simulink library "ctrlAllocMatrix_cl"  (R2018b)
settings: Solver=VariableStepAuto  StartTime=0.0  StopTime=10.0  RelTol=1e-3
undefined symbols (not defined in the file or in its folder): aeroStruct
libraries: vrlib x3, vectorNormalizer_ul x2, linearLeastSqrs_ul x1, dynamicPressure_ul x1, alphaBeta_ul x1, localApparentWind_ul x1
settings Model: Creator=mcobb  LastModifiedBy=James Reed

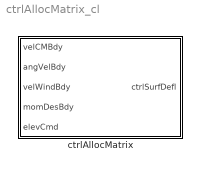
== system ctrlAllocMatrix_cl ==
  ctrlAllocMatrix : Subsystem  mask{aeroStruct=aeroStruct, fluidDensity=0, ctrlUpMax=0, ctrlDnMax=0}
      mask prompts: aeroStruct "Aerodynamic surface structure"; fluidDensity "Fluid density"; ctrlUpMax "Max Up Ctrl Surf Defl"; ctrlDnMax "Max Down Ctrl Surf Defl"
      mask TypeOptions aeroStruct: momentComponentVector/aeroStruct
      mask TypeOptions fluidDensity: momentComponentVector/fluidDensity

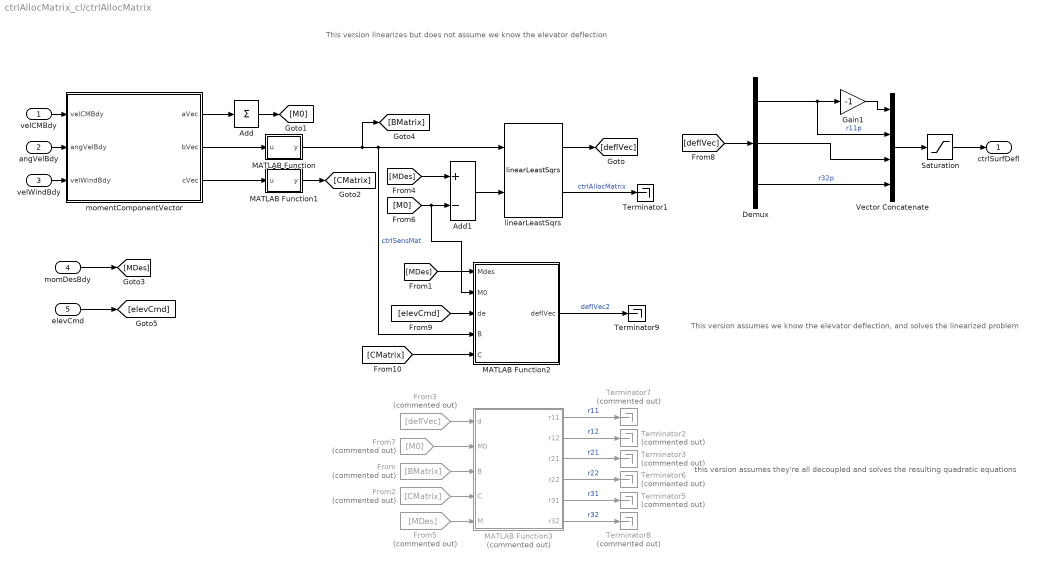
== system ctrlAllocMatrix_cl/ctrlAllocMatrix ==
  note: This version linearizes but does not assume we know the elevator deflection
  note: this version assumes they're all decoupled and solves the resulting quadratic equations
  note: This version assumes we know the elevator deflection, and solves the linearized problem
  velCMBdy : Inport
  angVelBdy : Inport  Port=2
  velWindBdy : Inport  Port=3
  momDesBdy : Inport  Port=4
  elevCmd : Inport  Port=5
  Add : Sum  Inputs=+  CollapseMode=Specified dimension  CollapseDim=2
  Add1 : Sum  Inputs=+-
  Demux : Demux  Outputs=3
  From : From  Commented=on  GotoTag=BMatrix
  From2 : From  Commented=on  GotoTag=CMatrix
  From3 : From  Commented=on  GotoTag=deflVec
  From5 : From  Commented=on  GotoTag=MDes
  From7 : From  Commented=on  GotoTag=M0
  Gain1 : Gain  Gain=-1
  MATLAB Function : MATLAB Function  TreatAsAtomicUnit=on
  MATLAB Function1 : MATLAB Function  TreatAsAtomicUnit=on
  MATLAB Function2 : MATLAB Function  TreatAsAtomicUnit=on
  MATLAB Function3 : MATLAB Function  Commented=on  TreatAsAtomicUnit=on
  Saturation : Saturate  UpperLimit=ctrlUpMax  LowerLimit=ctrlDnMax
  Terminator1 : Terminator
  Terminator{2..3,5..8} (6 alike) : Terminator  Commented=on
  Terminator9 : Terminator
  Vector Concatenate : Concatenate  NumInputs=4
  linearLeastSqrs : linearLeastSqrs_ul/linearLeastSqrs  SystemSampleTime=-1
  momentComponentVector : Subsystem  mask{aeroStruct=aeroStruct, fluidDensity=fluidDensity}
      mask prompts: aeroStruct "Aerodynamic surface structure"; fluidDensity "Fluid density"
      mask help:
      | Input must be an 1×N struct array with fields:
      |     refArea
      |     aeroCentPosVec
      |     spanUnitVec
      |     chordUnitVec
      |     CL
      |     CD
      |     alpha
      |     GainCL
      |     GainCD
      |
      | where N is the number of aerodynamic surfaces
  ctrlSurfDefl : Outport
  wires:
  velWindBdy/1 -> momentComponentVector/3(velWindBdy)
  velCMBdy/1 -> momentComponentVector/1(velCMBdy)
  angVelBdy/1 -> momentComponentVector/2(angVelBdy)
  momentComponentVector/1(aVec) -> Add/1
  momentComponentVector/3(cVec) -> MATLAB Function1/1(u)
  Add/1 -> [M0]
  momDesBdy/1 -> [MDes]
  [M0] -> MATLAB Function2/2(M0), Add1/2
  Add1/1 -> linearLeastSqrs/2
  MATLAB Function/1(y) -> [BMatrix], MATLAB Function2/4(B), linearLeastSqrs/1  "ctrlSensMat"
  linearLeastSqrs/1 -> [deflVec]
  momentComponentVector/2(bVec) -> MATLAB Function/1(u)
  Demux/2 -> Vector Concatenate/3
  Demux/1 -> Vector Concatenate/2, Gain1/1  "r11p"
  Vector Concatenate/1 -> Saturation/1
  Saturation/1 -> ctrlSurfDefl/1
  Gain1/1 -> Vector Concatenate/1
  linearLeastSqrs/2 -> Terminator1/1  "ctrlAllocMatrix"
  MATLAB Function1/1(y) -> [CMatrix]
  [MDes] -> Add1/1
  Demux/3 -> Vector Concatenate/4  "r32p"
  From2/1 -> MATLAB Function3/4(C)
  From3/1 -> MATLAB Function3/1(d)
  From5/1 -> MATLAB Function3/5(M)
  From7/1 -> MATLAB Function3/2(M0)
  From/1 -> MATLAB Function3/3(B)
  MATLAB Function3/2(r12) -> Terminator2/1  "r12"
  MATLAB Function3/3(r21) -> Terminator3/1  "r21"
  MATLAB Function3/5(r31) -> Terminator5/1  "r31"
  MATLAB Function3/6(r32) -> Terminator8/1  "r32"
  MATLAB Function3/4(r22) -> Terminator6/1  "r22"
  MATLAB Function3/1(r11) -> Terminator7/1  "r11"
  elevCmd/1 -> [elevCmd]
  [MDes] -> MATLAB Function2/1(Mdes)
  [elevCmd] -> MATLAB Function2/3(de)
  [CMatrix] -> MATLAB Function2/5(C)
  MATLAB Function2/1(deflVec) -> Terminator9/1  "deflVec2"
  [deflVec] -> Demux/1

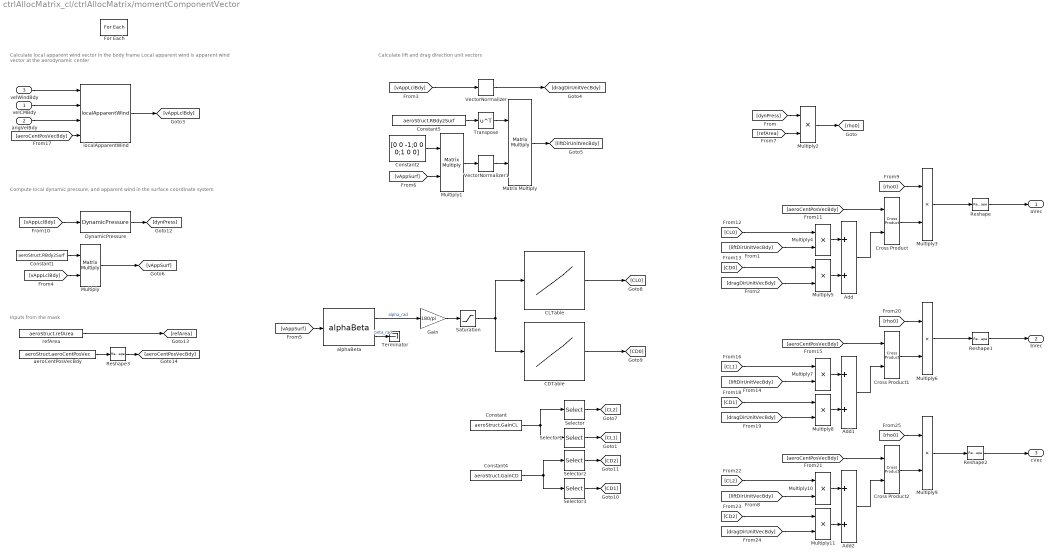
== system ctrlAllocMatrix_cl/ctrlAllocMatrix/momentComponentVector ==
  note: Compute local dynamic pressure,
      | and apparent wind in the surface coordinate system
  note: Inputs from the mask
  note: Calculate lift and drag direction unit vectors
  note: Calculate local apparent wind vector in the body frame
      | Local apparent wind is apparent wind vector at the aerodynamic center
  velCMBdy : Inport
  angVelBdy : Inport  Port=2
  velWindBdy : Inport  Port=3
  Add : Sum
  Add1 : Sum
  Add2 : Sum
  CDTable : Lookup_n-D  NumberOfTableDimensions=1  LookupTableObject=CLTable  BreakpointsForDimension1=aeroStruct.alpha  Table=aeroStruct.CD  ExtrapMethod=Clip  UseLastTableValue=on  InternalRulePriority=Speed  RndMeth=Simplest  InputSameDT=on
  CLTable : Lookup_n-D  NumberOfTableDimensions=1  LookupTableObject=CLTable  BreakpointsForDimension1=aeroStruct.alpha  Table=aeroStruct.CL  ExtrapMethod=Clip  UseLastTableValue=on  InternalRulePriority=Speed  RndMeth=Simplest  InputSameDT=on
  Constant : Constant  Value=aeroStruct.GainCL
  Constant1 : Constant  Value=aeroStruct.RBdy2Surf
  Constant2 : Constant  Value=[0 0 -1;0 0 0;1 0 0]
  Constant4 : Constant  Value=aeroStruct.GainCD
  Constant5 : Constant  Value=aeroStruct.RBdy2Surf
  Cross Product : vrlib/Utilities/Cross Product
      settings: SourceProductBaseCode=VR
  Cross Product1 : vrlib/Utilities/Cross Product
      settings: SourceProductBaseCode=VR
  Cross Product2 : vrlib/Utilities/Cross Product
      settings: SourceProductBaseCode=VR
  DynamicPressure : dynamicPressure_ul/DynamicPressure  rho=fluidDensity
  For Each : ForEach  DisableCoverage=on  IterateSubsysMaskParameter=on,off  SubsysMaskParameterIterationDimension=2,1  IndexMode=One-based
  Gain : Gain  Gain=180/pi
  Matrix Multiply : Product  Multiplication=Matrix(*)
  Multiply : Product  Multiplication=Matrix(*)
  Multiply1 : Product  Multiplication=Matrix(*)
  Multiply{2..11} (10 alike) : Product
  Reshape{,1..3} (4 alike) : Reshape  OutputDimensionality=Column vector (2-D)
  Saturation : Saturate  UpperLimit=90  LowerLimit=-90
  Selector : Selector  InputPortWidth=3  IndexOptions=Index vector (dialog)  Indices=1  OutputSizes=1
  Selector1 : Selector  InputPortWidth=3  IndexOptions=Index vector (dialog)  Indices=2  OutputSizes=1
  Selector2 : Selector  InputPortWidth=3  IndexOptions=Index vector (dialog)  Indices=1  OutputSizes=1
  Selector3 : Selector  InputPortWidth=3  IndexOptions=Index vector (dialog)  Indices=2  OutputSizes=1
  Terminator : Terminator
  Transpose : Math  Operator=transpose  SaturateOnIntegerOverflow=on
  "VectorNormalizer " : vectorNormalizer_ul/VectorNormalizer   SystemSampleTime=-1
  VectorNormalizer1 : vectorNormalizer_ul/VectorNormalizer   SystemSampleTime=-1
  aeroCentPosVecBdy : Constant  Value=aeroStruct.aeroCentPosVec
  alphaBeta : alphaBeta_ul/alphaBeta  SystemSampleTime=-1
  localApparentWind : localApparentWind_ul/localApparentWind  SystemSampleTime=-1
  refArea : Constant  Value=aeroStruct.refArea
  aVec : Outport  PortDimensions=[3 1]  ConcatenationDimension=2
  bVec : Outport  Port=2  PortDimensions=[3 1]  ConcatenationDimension=2
  cVec : Outport  Port=3  PortDimensions=[3 1]  ConcatenationDimension=2
  wires:
  velWindBdy/1 -> localApparentWind/1
  [vAppLclBdy] -> "VectorNormalizer "/1
  "VectorNormalizer "/1 -> [dragDirUnitVecBdy]
  Constant1/1 -> Multiply/1
  [vAppLclBdy] -> Multiply/2
  Multiply/1 -> [vAppSurf]
  [vAppSurf] -> alphaBeta/1
  [vAppSurf] -> Multiply1/2
  Constant2/1 -> Multiply1/1
  Multiply1/1 -> VectorNormalizer1/1
  alphaBeta/2 -> Terminator/1  "beta_rad"
  CDTable/1 -> [CD0]
  DynamicPressure/1 -> [dynPress]
  [vAppLclBdy] -> DynamicPressure/1
  Constant5/1 -> Transpose/1
  Matrix Multiply/1 -> [liftDirUnitVecBdy]
  Transpose/1 -> Matrix Multiply/1
  VectorNormalizer1/1 -> Matrix Multiply/2
  aeroCentPosVecBdy/1 -> Reshape3/1
  refArea/1 -> [refArea]
  Reshape3/1 -> [aeroCentPosVecBdy]
  alphaBeta/1 -> Gain/1  "alpha_rad"
  velCMBdy/1 -> localApparentWind/2
  angVelBdy/1 -> localApparentWind/3
  [aeroCentPosVecBdy] -> localApparentWind/4
  localApparentWind/1 -> [vAppLclBdy]
  Gain/1 -> Saturation/1
  CLTable/1 -> [CL0]
  Saturation/1 -> CDTable/1, CLTable/1
  Constant/1 -> Selector/1, Selector1/1
  Selector1/1 -> [CL1]
  Selector/1 -> [CL2]
  Selector2/1 -> [CD2]
  Selector3/1 -> [CD1]
  Constant4/1 -> Selector2/1, Selector3/1
  [dynPress] -> Multiply2/1
  [refArea] -> Multiply2/2
  Multiply2/1 -> [rho0]
  [rho0] -> Multiply3/1
  Cross Product/1 -> Multiply3/2
  [aeroCentPosVecBdy] -> Cross Product/1
  Multiply3/1 -> Reshape/1
  Add/1 -> Cross Product/2
  Multiply4/1 -> Add/1
  Multiply5/1 -> Add/2
  [dragDirUnitVecBdy] -> Multiply5/2
  [liftDirUnitVecBdy] -> Multiply4/2
  [CL0] -> Multiply4/1
  [CD0] -> Multiply5/1
  [CD1] -> Multiply8/1
  [CL1] -> Multiply7/1
  [liftDirUnitVecBdy] -> Multiply7/2
  [dragDirUnitVecBdy] -> Multiply8/2
  Multiply8/1 -> Add1/2
  Multiply7/1 -> Add1/1
  Add1/1 -> Cross Product1/2
  Multiply6/1 -> Reshape1/1
  [aeroCentPosVecBdy] -> Cross Product1/1
  Cross Product1/1 -> Multiply6/2
  [rho0] -> Multiply6/1
  [rho0] -> Multiply9/1
  Cross Product2/1 -> Multiply9/2
  [aeroCentPosVecBdy] -> Cross Product2/1
  Multiply9/1 -> Reshape2/1
  Add2/1 -> Cross Product2/2
  Multiply10/1 -> Add2/1
  Multiply11/1 -> Add2/2
  [dragDirUnitVecBdy] -> Multiply11/2
  [liftDirUnitVecBdy] -> Multiply10/2
  [CL2] -> Multiply10/1
  [CD2] -> Multiply11/1
  Reshape/1 -> aVec/1
  Reshape1/1 -> bVec/1
  Reshape2/1 -> cVec/1

== matlab function ctrlAllocMatrix_cl/ctrlAllocMatrix/MATLAB Function1 ==
  data: u input; y output
function y = fcn(u)
y = [-u(:,1)+u(:,2) u(:,3:end)];

== matlab function ctrlAllocMatrix_cl/ctrlAllocMatrix/MATLAB Function ==
  data: u input; y output
function y = fcn(u)
y = [-u(:,1)+u(:,2) u(:,3:end)];

== matlab function ctrlAllocMatrix_cl/ctrlAllocMatrix/MATLAB Function2 ==
  data: Mdes input; deflVec output size=[1 3]; M0 input; de input; B input; C input
function deflVec = fcn(Mdes,M0,de,B,C)

M = Mdes(:)-M0(:) -B(:,2)*de - C(:,2)*de^2;

B0 = [B(:,1) B(:,3)];


d = inv(B0'*B0)*B0'*M(:);

deflVec = [d(1) de d(2)];

== matlab function ctrlAllocMatrix_cl/ctrlAllocMatrix/MATLAB Function3 ==
  data: d input; r11 output; r12 output; M0 input; B input; C input; M input; r21 output; r22 output; r31 output; r32 output
function [r11,r12,r21,r22,r31,r32] = fcn(d,M0,B,C,M)

a = diag(C);
b = diag(B);
c = M0(:)-M(:);

r = real([(-b+sqrt(b.^2-4*a.*c))./(2*a) (-b-sqrt(b.^2-4*a.*c))./(2*a)]);
r11 = r(1,1);
r12 = r(1,2);
r21 = r(2,1);
r22 = r(2,2);
r31 = r(3,1);
r32 = r(3,2);

% [r11,r12,r21,r22,r31,r32]
